simulink library "time_coord_rotations_lib"  (R2018b)
settings: Solver=VariableStepAuto  StartTime=0.0  StopTime=10.0  RelTol=1e-3
undefined symbols (not defined in the file): fswParams
libraries: coord_rotation_lib x1
settings Model: Creator=IvanMachuca  LastModifiedBy=aact_

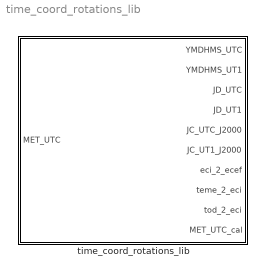
== system time_coord_rotations_lib ==
  time_coord_rotations_lib : Subsystem  TreatAsAtomicUnit=on  mask{time_offset=fswParams.sensors.time_offset}
      mask prompts: time_offset "Time error correction"
      mask TypeOptions time_offset: Constant1/Value

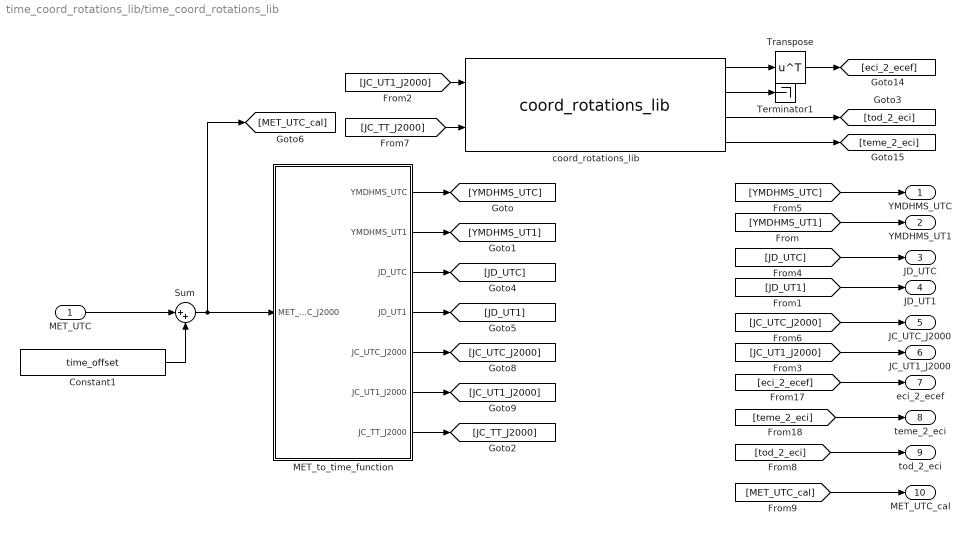
== system time_coord_rotations_lib/time_coord_rotations_lib ==
  "MET_UTC " : Inport
  Constant1 : Constant  Value=time_offset
  MET_to_time_function : MATLAB Function  TreatAsAtomicUnit=on
  Sum : Sum  Inputs=|++
  Terminator1 : Terminator
  Transpose : Math  Operator=transpose  SaturateOnIntegerOverflow=on
  coord_rotations_lib : coord_rotation_lib/coord_rotations_lib  SystemSampleTime=-1
  "YMDHMS_UTC " : Outport
  "YMDHMS_UT1 " : Outport  Port=2
  "JD_UTC " : Outport  Port=3
  JD_UT1 : Outport  Port=4
  "JC_UTC_J2000 " : Outport  Port=5
  JC_UT1_J2000 : Outport  Port=6
  "eci_2_ecef " : Outport  Port=7
  teme_2_eci : Outport  Port=8
  tod_2_eci : Outport  Port=9
  MET_UTC_cal : Outport  Port=10
  wires:
  [tod_2_eci] -> tod_2_eci/1
  coord_rotations_lib/2 -> Terminator1/1
  coord_rotations_lib/1 -> Transpose/1
  coord_rotations_lib/3 -> [tod_2_eci]
  [YMDHMS_UTC] -> "YMDHMS_UTC "/1
  [YMDHMS_UT1] -> "YMDHMS_UT1 "/1
  [JD_UTC] -> "JD_UTC "/1
  [JD_UT1] -> JD_UT1/1
  MET_to_time_function/5(JC_UTC_J2000) -> [JC_UTC_J2000]
  [JC_UTC_J2000] -> "JC_UTC_J2000 "/1
  MET_to_time_function/6(JC_UT1_J2000) -> [JC_UT1_J2000]
  [JC_UT1_J2000] -> coord_rotations_lib/1
  [JC_UT1_J2000] -> JC_UT1_J2000/1
  [JC_TT_J2000] -> coord_rotations_lib/2
  [eci_2_ecef] -> "eci_2_ecef "/1
  coord_rotations_lib/4 -> [teme_2_eci]
  [teme_2_eci] -> teme_2_eci/1
  MET_to_time_function/3(JD_UTC) -> [JD_UTC]
  MET_to_time_function/4(JD_UT1) -> [JD_UT1]
  MET_to_time_function/1(YMDHMS_UTC) -> [YMDHMS_UTC]
  MET_to_time_function/2(YMDHMS_UT1) -> [YMDHMS_UT1]
  MET_to_time_function/7(JC_TT_J2000) -> [JC_TT_J2000]
  Transpose/1 -> [eci_2_ecef]
  Sum/1 -> [MET_UTC_cal], MET_to_time_function/1(MET_UTC_J2000)
  "MET_UTC "/1 -> Sum/1
  Constant1/1 -> Sum/2
  [MET_UTC_cal] -> MET_UTC_cal/1

== matlab function time_coord_rotations_lib/MET_to_time_function ==
  data: MET_UTC_J2000 input double size=1; YMDHMS_UTC output double size=6; YMDHMS_UT1 output double size=6; JD_UTC output double size=1; JD_UT1 output double size=1; JC_UTC_J2000 output double size=1; JC_UT1_J2000 output double size=1; simParams parameter; JC_TT_J2000 output double size=1
function [YMDHMS_UTC,YMDHMS_UT1,JD_UTC,JD_UT1,JC_UTC_J2000,JC_UT1_J2000,JC_TT_J2000] = time_lib(MET_UTC_J2000,simParams)
%TIME_LIB 
% 
% Time conversions for SOC-i GNC software. Input is assumed to be the
% Mission Elapsed Time in seconds since the J2000 epoch in the UTC frame. 
%
% Devan Tormey & Taylor Reynolds
%#codegen

% OFFSETS FOR TIME FRAME CHANGE
DUT1        = simParams.time.DUT1;          % UTC -> UT1 offset
TAI_offset  = simParams.time.TAI_offset;    % UTC -> TAI offset
DTT_TAI     = simParams.time.DTT_TAI;       % TAI -> TT offset

% CONVERT INPUT UTC TO TAI, TT, and UT1
MET_TAI_J2000 = MET_UTC_J2000 + TAI_offset;
MET_TT_J2000  = MET_TAI_J2000 + DTT_TAI;
MET_UT1_J2000 = MET_UTC_J2000 + DUT1;

% convert the UTC time
[y,m,d,h,min,s,JC_UTC_J2000,JD_UTC] = jseconds2ymdhms(MET_UTC_J2000);
YMDHMS_UTC  = [ y; m; d; h; min; s ];

% convert the UT1 time
[y,m,d,h,min,s,JC_UT1_J2000,JD_UT1] = jseconds2ymdhms(MET_UT1_J2000);
YMDHMS_UT1  = [ y; m; d; h; min; s ];

% convert the TT time
[~,~,~,~,~,~,JC_TT_J2000,~] = jseconds2ymdhms(MET_TT_J2000);

end
